simulink model "LQR"  (R2021b)
settings: Solver=VariableStepAuto  StartTime=0.0  StopTime=5  RelTol=1e-3
values from neighbouring files (symbols this model uses):
  F = lqr(A,B,Q,R)    [simConstants.m]
  Td = 100e-6    (= 0.0001)    [simConstants.m]
libraries: simulink_extras x2
settings Model: Creator=logan  LastModifiedBy=logan

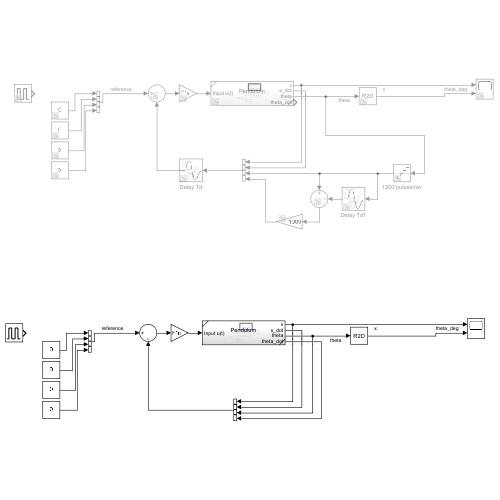
[thumbnail: Simulink's stored preview of the top-level diagram]
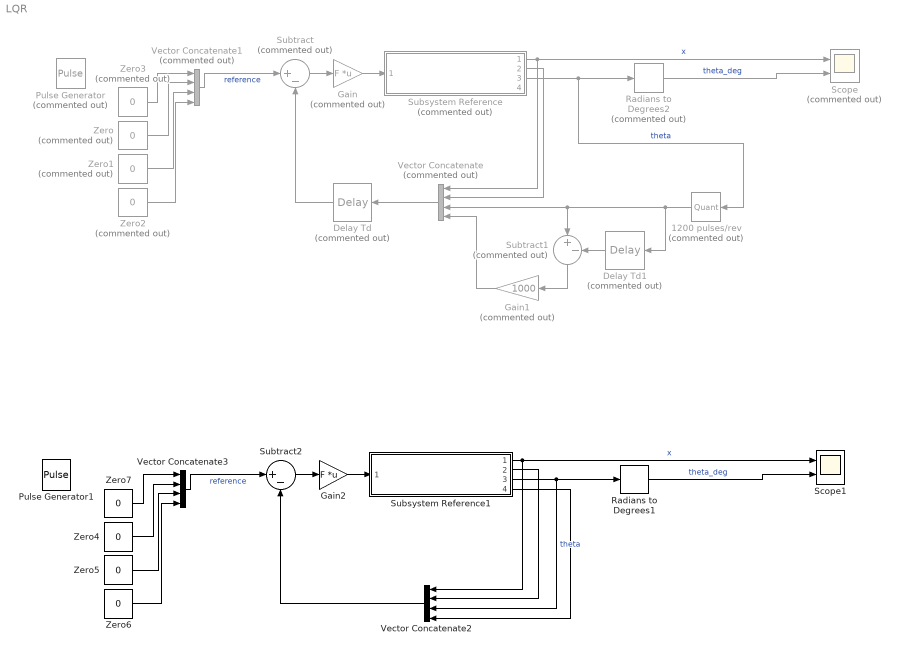
== system LQR ==
  1200 pulses/rev : Quantizer  Commented=on  QuantizationInterval=(2*pi)/1200
  Delay Td : TransportDelay  Commented=on  DelayTime=Td*10
  Delay Td1 : TransportDelay  Commented=on  DelayTime=1e-3
  Gain : Gain  Commented=on  Gain=F  Multiplication=Matrix(K*u)
  Gain1 : Gain  Commented=on  Gain=1000
  Gain2 : Gain  Gain=F  Multiplication=Matrix(K*u)
  Pulse Generator : DiscretePulseGenerator  Commented=on  PulseType=Time based  Period=20  PulseWidth=50
  Pulse Generator1 : DiscretePulseGenerator  PulseType=Time based  Period=20  PulseWidth=50
  Radians to Degrees1 : simulink_extras/Transformations/Radians to Degrees
  Radians to Degrees2 : simulink_extras/Transformations/Radians to Degrees  Commented=on
  Scope : Scope  Commented=on  NumInputPorts=2
  Scope1 : Scope  NumInputPorts=2
  Subsystem Reference : Subsystem  Commented=on  ReferencedSubsystem=Pendulum
  Subsystem Reference1 : Subsystem  ReferencedSubsystem=Pendulum
  Subtract : Sum  Commented=on  Inputs=|+-
  Subtract1 : Sum  Commented=on  Inputs=|+-
  Subtract2 : Sum  Inputs=|+-
  Vector Concatenate : Concatenate  Commented=on  NumInputs=4
  Vector Concatenate1 : Concatenate  Commented=on  NumInputs=4
  Vector Concatenate2 : Concatenate  NumInputs=4
  Vector Concatenate3 : Concatenate  NumInputs=4
  Zero{,1..3} (4 alike) : Constant  Commented=on  Value=0  OutDataTypeStr=Inherit: Inherit via back propagation
  Zero{4..7} (4 alike) : Constant  Value=0  OutDataTypeStr=Inherit: Inherit via back propagation
  wires:
  Subtract/1 -> Gain/1
  Vector Concatenate1/1 -> Subtract/1  "reference"
  Subsystem Reference/3 -> 1200 pulses/rev/1, Radians to Degrees2/1  "theta"
  Radians to Degrees2/1 -> Scope/2  "theta_deg"
  Subsystem Reference/1 -> Scope/1, Vector Concatenate/1  "x"
  Vector Concatenate/1 -> Delay Td/1
  Delay Td/1 -> Subtract/2
  Gain/1 -> Subsystem Reference/1
  Zero/1 -> Vector Concatenate1/2
  Zero1/1 -> Vector Concatenate1/3
  Zero2/1 -> Vector Concatenate1/4
  Zero3/1 -> Vector Concatenate1/1
  1200 pulses/rev/1 -> Delay Td1/1, Vector Concatenate/3, Subtract1/1
  Delay Td1/1 -> Subtract1/2
  Subtract1/1 -> Gain1/1
  Subsystem Reference/2 -> Vector Concatenate/2
  Gain1/1 -> Vector Concatenate/4
  Zero5/1 -> Vector Concatenate3/3
  Zero7/1 -> Vector Concatenate3/1
  Zero6/1 -> Vector Concatenate3/4
  Vector Concatenate3/1 -> Subtract2/1  "reference"
  Subsystem Reference1/1 -> Scope1/1, Vector Concatenate2/1  "x"
  Radians to Degrees1/1 -> Scope1/2  "theta_deg"
  Subtract2/1 -> Gain2/1
  Subsystem Reference1/3 -> Radians to Degrees1/1, Vector Concatenate2/3  "theta"
  Vector Concatenate2/1 -> Subtract2/2
  Zero4/1 -> Vector Concatenate3/2
  Gain2/1 -> Subsystem Reference1/1
  Subsystem Reference1/2 -> Vector Concatenate2/2
  Subsystem Reference1/4 -> Vector Concatenate2/4
